simulink model "sm_wing_landing_gear"  (R2021b)
settings: Solver=ode45  StartTime=0  StopTime=10  RelTol=1e-4  AbsTol=1e-4  EnableMultiTasking=on
model workspace (MAT data in the model file):
  ddgrey = [0.15 0.15 0.15]
  dgrey = [0.3 0.3 0.3]
  grey = [0.5 0.5 0.5]
  lgrey = [0.7 0.7 0.7]
  rho_alum = 2700
undefined symbols (not defined in the file): sigbuilder_block, X, Y, Z
libraries: sm_lib x59, sm_wing_landing_gear_lib x45, nesl_utility x7, simulink x2
(part 3 of 3)

== system sm_wing_landing_gear/Wing Landing Gear/Main Column/Main Column/Art Links Bracket Housing ==
  Annular Cylinder : sm_wing_landing_gear_lib/Annular Cylinder  Ro=Ro  Ri=Ri  L=L  rho=rho  clr=clr  opc=1
      settings: SourceProductBaseCode=MS
  Left Side Transform : sm_lib/Frames and Transforms/Rigid Transform  TranslationMethod=Cylindrical  TranslationStandardOffset=0  TranslationLengthUnit=cm  TranslationStandardAxis=-Y  TranslationCartesianOffset=[0 0 0]  TranslationROffset=Ro  TranslationROffsetUnits=cm  TranslationZOffset=L/2  TranslationZOffsetUnits=cm  TranslationThetaOffset=-90  TranslationThetaOffsetUnits=deg  RotationMethod=AlignedAxes  RotationAngleUnits=deg  RotationStandardAxis=+Z  RotationAngle=0  RotationArbitraryAxis=[0 0 1]  FollAlignAxisA=+X  BaseAlignAxisA=-Y  FollAlignAxisB=+Y  BaseAlignAxisB=+X  RotationSequenceAxes=FollowerAxes  RotationSequence=XYX  RotationSequenceAngles=[0 0 0]  RotationSequenceAnglesUnits=deg  RotationMatrix=[1 0 0; 0 1 0; 0 0 1]
  Right Side Transform : sm_lib/Frames and Transforms/Rigid Transform  TranslationMethod=Cylindrical  TranslationStandardOffset=0  TranslationLengthUnit=cm  TranslationStandardAxis=-Y  TranslationCartesianOffset=[0 0 0]  TranslationROffset=Ro  TranslationROffsetUnits=cm  TranslationZOffset=L/2  TranslationZOffsetUnits=cm  TranslationThetaOffset=90  TranslationThetaOffsetUnits=deg  RotationMethod=AlignedAxes  RotationAngleUnits=deg  RotationStandardAxis=+Z  RotationAngle=0  RotationArbitraryAxis=[0 0 1]  FollAlignAxisA=+X  BaseAlignAxisA=+Y  FollAlignAxisB=+Y  BaseAlignAxisB=-X  RotationSequenceAxes=FollowerAxes  RotationSequence=XYX  RotationSequenceAngles=[0 0 0]  RotationSequenceAnglesUnits=deg  RotationMatrix=[1 0 0; 0 1 0; 0 0 1]
  T : PMIOPort  Side=Right
  L : PMIOPort  Port=2  Side=Left
  B : PMIOPort  Port=3  Side=Left
  R : PMIOPort  Port=4  Side=Left
  connections:
  Left Side Transform/RConn1 -- L/RConn1
  T/RConn1 -- Annular Cylinder/RConn1
  Right Side Transform/RConn1 -- R/RConn1
  Left Side Transform/LConn1 -- Right Side Transform/LConn1 -- Annular Cylinder/LConn1 -- B/RConn1

== system sm_wing_landing_gear/Wing Landing Gear/Main Column/Main Column/Main Actuator Bracket Housing ==
  Annular Cylinder : sm_wing_landing_gear_lib/Annular Cylinder  Ro=Ro  Ri=Ri  L=L  rho=rho  clr=clr  opc=1
      settings: SourceProductBaseCode=MS
  Left Side Transform : sm_lib/Frames and Transforms/Rigid Transform  TranslationMethod=Cylindrical  TranslationStandardOffset=0  TranslationLengthUnit=cm  TranslationStandardAxis=-Y  TranslationCartesianOffset=[0 0 0]  TranslationROffset=Ro  TranslationROffsetUnits=cm  TranslationZOffset=L/2  TranslationZOffsetUnits=cm  TranslationThetaOffset=180  TranslationThetaOffsetUnits=deg  RotationMethod=AlignedAxes  RotationAngleUnits=deg  RotationStandardAxis=+Z  RotationAngle=0  RotationArbitraryAxis=[0 0 1]  FollAlignAxisA=+X  BaseAlignAxisA=-X  FollAlignAxisB=+Y  BaseAlignAxisB=-Y  RotationSequenceAxes=FollowerAxes  RotationSequence=XYX  RotationSequenceAngles=[0 0 0]  RotationSequenceAnglesUnits=deg  RotationMatrix=[1 0 0; 0 1 0; 0 0 1]
  Right Side Transform : sm_lib/Frames and Transforms/Rigid Transform  TranslationMethod=Cylindrical  TranslationStandardOffset=0  TranslationLengthUnit=cm  TranslationStandardAxis=-Y  TranslationCartesianOffset=[0 0 0]  TranslationROffset=Ro  TranslationROffsetUnits=cm  TranslationZOffset=L/2  TranslationZOffsetUnits=cm  TranslationThetaOffset=0  TranslationThetaOffsetUnits=deg  RotationMethod=None  RotationAngleUnits=deg  RotationStandardAxis=+Z  RotationAngle=0  RotationArbitraryAxis=[0 0 1]  FollAlignAxisA=+X  BaseAlignAxisA=+Y  FollAlignAxisB=+Y  BaseAlignAxisB=-X  RotationSequenceAxes=FollowerAxes  RotationSequence=XYX  RotationSequenceAngles=[0 0 0]  RotationSequenceAnglesUnits=deg  RotationMatrix=[1 0 0; 0 1 0; 0 0 1]
  T : PMIOPort  Side=Right
  L : PMIOPort  Port=2  Side=Left
  B : PMIOPort  Port=3  Side=Left
  R : PMIOPort  Port=4  Side=Left
  connections:
  B/RConn1 -- Annular Cylinder/LConn1 -- Right Side Transform/LConn1 -- Left Side Transform/LConn1
  Right Side Transform/RConn1 -- R/RConn1
  T/RConn1 -- Annular Cylinder/RConn1
  Left Side Transform/RConn1 -- L/RConn1

== system sm_wing_landing_gear/Wing Landing Gear/Main Column/Main Column/Main Column Bottom Cylinder ==
  Annular Cylinder : sm_wing_landing_gear_lib/Annular Cylinder  Ro=Ro  Ri=Ri  L=L  rho=rho  clr=clr  opc=1
      settings: SourceProductBaseCode=MS
  Side Transform : sm_lib/Frames and Transforms/Rigid Transform  TranslationMethod=Cylindrical  TranslationStandardOffset=0  TranslationLengthUnit=cm  TranslationStandardAxis=+X  TranslationCartesianOffset=[ 0 0]  TranslationROffset=Ro  TranslationROffsetUnits=cm  TranslationZOffset=Oh  TranslationZOffsetUnits=cm  TranslationThetaOffset=Ah  TranslationThetaOffsetUnits=deg  RotationMethod=StandardAxis  RotationAngleUnits=deg  RotationStandardAxis=+Z  RotationAngle=Ah  RotationArbitraryAxis=[0 0 1]  FollAlignAxisA=+X  BaseAlignAxisA=+Y  FollAlignAxisB=+Y  BaseAlignAxisB=+Z  RotationSequenceAxes=FollowerAxes  RotationSequence=XYX  RotationSequenceAngles=[0 0 0]  RotationSequenceAnglesUnits=deg  RotationMatrix=[1 0 0; 0 1 0; 0 0 1]
  B : PMIOPort  Side=Left
  T : PMIOPort  Port=2  Side=Right
  D : PMIOPort  Port=3  Side=Left
  connections:
  Side Transform/LConn1 -- Annular Cylinder/LConn1 -- B/RConn1
  Annular Cylinder/RConn1 -- T/RConn1
  Side Transform/RConn1 -- D/RConn1

== system sm_wing_landing_gear/Wing Landing Gear/Main Column/Main Column/Main Column Top Cylinder ==
  Annular Cylinder : sm_wing_landing_gear_lib/Annular Cylinder  Ro=Ro  Ri=Ri  L=L  rho=rho  clr=clr  opc=1
      settings: SourceProductBaseCode=MS
  B : PMIOPort  Side=Left
  T : PMIOPort  Port=2  Side=Right
  connections:
  Annular Cylinder/RConn1 -- T/RConn1
  B/RConn1 -- Annular Cylinder/LConn1

== system sm_wing_landing_gear/Wing Landing Gear/Main Column/Main Column/Piston  ==
  Flange : sm_wing_landing_gear_lib/Annular Cylinder  Ro=Rf  Ri=Ri  L=Tf  rho=rho_alum  clr=clr  opc=1
      settings: SourceProductBaseCode=MS
  Piston : sm_wing_landing_gear_lib/Annular Cylinder  Ro=Ro  Ri=Ri  L=L  rho=rho_alum  clr=clr  opc=1
      settings: SourceProductBaseCode=MS
  B : PMIOPort  Side=Right
  T : PMIOPort  Port=2  Side=Left
  connections:
  B/RConn1 -- Flange/LConn1
  Piston/RConn1 -- T/RConn1
  Flange/RConn1 -- Piston/LConn1

== system sm_wing_landing_gear/Wing Landing Gear/Main Column/Main Column/Spherical Cup and Holder ==
  Cup : Subsystem  mask{Rb=Rci, Ro=Rco, T=2, A=210, Cc=cclr}
      mask prompts: Rb "Ball radius:"; Ro "Cup outer radius:"; T "Strip thickness:"; A "Cup angle:"; Cc "Color:"
      mask init:
      | theta = (linspace(-(A/2+90),(A/2-90),A+1)*pi/180)';
      | cup_profile = [Ro*cos(theta) Ro*sin(theta)];
      | theta = (linspace((A/2-90),-(A/2+90),A+1)*pi/180)';
      | cup_profile = vertcat(cup_profile,[Rb*cos(theta) Rb*sin(theta)]);
  Holder Half A : sm_lib/Body Elements/Extruded Solid  GraphicAmbientColor=[0.5 0.0 0.0 1.0]  BasedOnType=Density  CenterOfMass=[0 0 0]  CenterOfMassUnits=m  GraphicDiffuseColor=hclr  ExportConvexHullGeometry=off  ExtrusionCrossSection=hinge_sec_a  ExtrusionCrossSectionUnits=cm  Density=rho  DensityUnits=kg/(m^3)  DoExposeReferenceFrame=on  GraphicEmissiveColor=[0.0 0.0 0.0 1.0]  ExportEntireGeometry=off  ExtrusionLength=Hh  ExtrusionLengthUnits=cm  ExtrusionType=General  SerializedFrames=<Frames/>  MarkerShape=Sphere  MarkerSize=10  GraphicType=FromGeometry  InertiaType=CalculateFromGeometry  Mass=1  MassUnits=kg  MomentsOfInertia=[1 1 1]  MomentsOfInertiaUnits=kg*m^2  PolygonNumSides=3  GraphicOpacity=1.0  PolygonOuterRadius=1  PolygonOuterRadiusUnits=m  ProductsOfInertia=[0 0 0]  ProductsOfInertiaUnits=kg*m^2  GraphicShininess=75  GraphicSpecularColor=[0.5 0.5 0.5 1.0]  GraphicVisPropType=SimpleVisualProperties
  Holder Half B : sm_lib/Body Elements/Extruded Solid  GraphicAmbientColor=[0.5 0.0 0.0 1.0]  BasedOnType=Density  CenterOfMass=[0 0 0]  CenterOfMassUnits=m  GraphicDiffuseColor=hclr  ExportConvexHullGeometry=off  ExtrusionCrossSection=hinge_sec_b  ExtrusionCrossSectionUnits=cm  Density=rho  DensityUnits=kg/(m^3)  DoExposeReferenceFrame=on  GraphicEmissiveColor=[0.0 0.0 0.0 1.0]  ExportEntireGeometry=off  ExtrusionLength=Hh  ExtrusionLengthUnits=cm  ExtrusionType=General  SerializedFrames=<Frames/>  MarkerShape=Sphere  MarkerSize=10  GraphicType=FromGeometry  InertiaType=CalculateFromGeometry  Mass=1  MassUnits=kg  MomentsOfInertia=[1 1 1]  MomentsOfInertiaUnits=kg*m^2  PolygonNumSides=3  GraphicOpacity=1.0  PolygonOuterRadius=1  PolygonOuterRadiusUnits=m  ProductsOfInertia=[0 0 0]  ProductsOfInertiaUnits=kg*m^2  GraphicShininess=75  GraphicSpecularColor=[0.5 0.5 0.5 1.0]  GraphicVisPropType=SimpleVisualProperties
  Holder-Cup Transform : sm_lib/Frames and Transforms/Rigid Transform  TranslationMethod=Cartesian  TranslationStandardOffset=0  TranslationLengthUnit=cm  TranslationStandardAxis=+X  TranslationCartesianOffset=[Oh 0 Hh/2]  TranslationROffset=0  TranslationROffsetUnits=m  TranslationZOffset=0  TranslationZOffsetUnits=m  TranslationThetaOffset=0  TranslationThetaOffsetUnits=deg  RotationMethod=None  RotationAngleUnits=deg  RotationStandardAxis=+Z  RotationAngle=0  RotationArbitraryAxis=[0 0 1]  FollAlignAxisA=+X  BaseAlignAxisA=+Y  FollAlignAxisB=+Y  BaseAlignAxisB=+Z  RotationSequenceAxes=FollowerAxes  RotationSequence=XYX  RotationSequenceAngles=[0 0 0]  RotationSequenceAnglesUnits=deg  RotationMatrix=[1 0 0; 0 1 0; 0 0 1]
  S : PMIOPort  Side=Right
  B : PMIOPort  Port=2  Side=Left
  connections:
  B/RConn1 -- Holder Half A/RConn1 -- Holder-Cup Transform/LConn1 -- Holder Half B/RConn1
  Holder-Cup Transform/RConn1 -- Cup/LConn1
  Cup/RConn1 -- S/RConn1

== system sm_wing_landing_gear/Wing Landing Gear/Main Column Locking Mechanism/Side Stay Linkage/Peg and Ball ==
  Ball : sm_lib/Body Elements/Spherical Solid  GraphicAmbientColor=[0.5 0.0 0.0 1.0]  BasedOnType=Density  CenterOfMass=[0 0 0]  CenterOfMassUnits=m  GraphicDiffuseColor=clr  Density=rho  DensityUnits=kg/(m^3)  DoExposeReferenceFrame=on  GraphicEmissiveColor=[0.0 0.0 0.0 1.0]  ExportEntireGeometry=off  SerializedExposedGeometries=<ExposedGeometries/>  SerializedFrames=<Frames/>  MarkerShape=Sphere  MarkerSize=10  GraphicType=FromGeometry  InertiaType=CalculateFromGeometry  Mass=1  MassUnits=kg  MomentsOfInertia=[1 1 1]  MomentsOfInertiaUnits=kg*m^2  GraphicOpacity=1.0  ProductsOfInertia=[0 0 0]  ProductsOfInertiaUnits=kg*m^2  GraphicShininess=75  GraphicSpecularColor=[0.5 0.5 0.5 1.0]  SphereRadius=Rb  SphereRadiusUnits=cm  GraphicVisPropType=SimpleVisualProperties
  Base-Peg Transform : sm_lib/Frames and Transforms/Rigid Transform  TranslationMethod=StandardAxis  TranslationStandardOffset=Lp/2  TranslationLengthUnit=cm  TranslationStandardAxis=+Z  TranslationCartesianOffset=[0 0 0]  TranslationROffset=0  TranslationROffsetUnits=m  TranslationZOffset=0  TranslationZOffsetUnits=m  TranslationThetaOffset=0  TranslationThetaOffsetUnits=deg  RotationMethod=None  RotationAngleUnits=deg  RotationStandardAxis=+Z  RotationAngle=0  RotationArbitraryAxis=[0 0 1]  FollAlignAxisA=+Z  BaseAlignAxisA=+X  FollAlignAxisB=+X  BaseAlignAxisB=-Z  RotationSequenceAxes=FollowerAxes  RotationSequence=XYX  RotationSequenceAngles=[0 0 0]  RotationSequenceAnglesUnits=deg  RotationMatrix=[1 0 0; 0 1 0; 0 0 1]
  Peg : sm_lib/Body Elements/Cylindrical Solid  GraphicAmbientColor=[0.5 0.0 0.0 1.0]  BasedOnType=Density  CenterOfMass=[0 0 0]  CenterOfMassUnits=m  GraphicDiffuseColor=clr  CylinderLength=Lp  CylinderLengthUnits=cm  CylinderRadius=Rp  CylinderRadiusUnits=cm  Density=rho  DensityUnits=kg/(m^3)  DoExposeReferenceFrame=on  GraphicEmissiveColor=[0.0 0.0 0.0 1.0]  ExportEntireGeometry=off  SerializedFrames=<Frames/>  MarkerShape=Sphere  MarkerSize=10  GraphicType=FromGeometry  InertiaType=CalculateFromGeometry  Mass=1  MassUnits=kg  MomentsOfInertia=[1 1 1]  MomentsOfInertiaUnits=kg*m^2  GraphicOpacity=1.0  ProductsOfInertia=[0 0 0]  ProductsOfInertiaUnits=kg*m^2  GraphicShininess=75  GraphicSpecularColor=[0.5 0.5 0.5 1.0]  GraphicVisPropType=SimpleVisualProperties
  Peg-Ball Transform : sm_lib/Frames and Transforms/Rigid Transform  TranslationMethod=StandardAxis  TranslationStandardOffset=Lp/2  TranslationLengthUnit=cm  TranslationStandardAxis=+Z  TranslationCartesianOffset=[0 0 0]  TranslationROffset=0  TranslationROffsetUnits=m  TranslationZOffset=0  TranslationZOffsetUnits=m  TranslationThetaOffset=0  TranslationThetaOffsetUnits=deg  RotationMethod=None  RotationAngleUnits=deg  RotationStandardAxis=+Z  RotationAngle=0  RotationArbitraryAxis=[0 0 1]  FollAlignAxisA=+Z  BaseAlignAxisA=+X  FollAlignAxisB=+X  BaseAlignAxisB=-Z  RotationSequenceAxes=FollowerAxes  RotationSequence=XYX  RotationSequenceAngles=[0 0 0]  RotationSequenceAnglesUnits=deg  RotationMatrix=[1 0 0; 0 1 0; 0 0 1]
  F : PMIOPort  Side=Right
  B : PMIOPort  Port=2  Side=Left
  connections:
  Base-Peg Transform/LConn1 -- B/RConn1
  Ball/RConn1 -- F/RConn1 -- Peg-Ball Transform/RConn1
  Base-Peg Transform/RConn1 -- Peg-Ball Transform/LConn1 -- Peg/RConn1

== system sm_wing_landing_gear/Wing Landing Gear/Main Column/Main Column/Spherical Cup and Holder/Cup ==
  Base-Center Transform : sm_lib/Frames and Transforms/Rigid Transform  TranslationMethod=StandardAxis  TranslationStandardOffset=Ro  TranslationLengthUnit=cm  TranslationStandardAxis=+Z  TranslationCartesianOffset=[0 0 0]  TranslationROffset=[]  TranslationROffsetUnits=m  TranslationZOffset=[]  TranslationZOffsetUnits=m  TranslationThetaOffset=[]  TranslationThetaOffsetUnits=deg  RotationMethod=None  RotationAngleUnits=deg  RotationStandardAxis=+X  RotationAngle=[]  RotationArbitraryAxis=[]  FollAlignAxisA=+X  BaseAlignAxisA=+Y  FollAlignAxisB=+Y  BaseAlignAxisB=+Z  RotationSequenceAxes=FollowerAxes  RotationSequence=XYX  RotationSequenceAngles=[0 0 0]  RotationSequenceAnglesUnits=deg  RotationMatrix=[1 0 0; 0 1 0; 0 0 1]
  Center-Strip A Transform : sm_lib/Frames and Transforms/Rigid Transform  TranslationMethod=None  TranslationStandardOffset=0  TranslationLengthUnit=m  TranslationStandardAxis=+X  TranslationCartesianOffset=[0 0 0]  TranslationROffset=[]  TranslationROffsetUnits=m  TranslationZOffset=[]  TranslationZOffsetUnits=m  TranslationThetaOffset=[]  TranslationThetaOffsetUnits=deg  RotationMethod=AlignedAxes  RotationAngleUnits=deg  RotationStandardAxis=+X  RotationAngle=[]  RotationArbitraryAxis=[]  FollAlignAxisA=+Y  BaseAlignAxisA=+Z  FollAlignAxisB=+Z  BaseAlignAxisB=-Y  RotationSequenceAxes=FollowerAxes  RotationSequence=XYX  RotationSequenceAngles=[0 0 0]  RotationSequenceAnglesUnits=deg  RotationMatrix=[1 0 0; 0 1 0; 0 0 1]
  Center-Strip B Transform : sm_lib/Frames and Transforms/Rigid Transform  TranslationMethod=None  TranslationStandardOffset=0  TranslationLengthUnit=m  TranslationStandardAxis=+X  TranslationCartesianOffset=[0 0 0]  TranslationROffset=[]  TranslationROffsetUnits=m  TranslationZOffset=[]  TranslationZOffsetUnits=m  TranslationThetaOffset=[]  TranslationThetaOffsetUnits=deg  RotationMethod=AlignedAxes  RotationAngleUnits=deg  RotationStandardAxis=+X  RotationAngle=[]  RotationArbitraryAxis=[]  FollAlignAxisA=+Z  BaseAlignAxisA=+X  FollAlignAxisB=+Y  BaseAlignAxisB=+Z  RotationSequenceAxes=FollowerAxes  RotationSequence=XYX  RotationSequenceAngles=[0 0 0]  RotationSequenceAnglesUnits=deg  RotationMatrix=[1 0 0; 0 1 0; 0 0 1]
  Cup Strip A : sm_lib/Body Elements/Extruded Solid  GraphicAmbientColor=[0.5 0.0 0.0 1.0]  BasedOnType=Density  CenterOfMass=[]  CenterOfMassUnits=m  GraphicDiffuseColor=Cc  ExportConvexHullGeometry=off  ExtrusionCrossSection=cup_profile  ExtrusionCrossSectionUnits=cm  Density=rho  DensityUnits=kg/(m^3)  DoExposeReferenceFrame=on  GraphicEmissiveColor=[0.0 0.0 0.0 1.0]  ExportEntireGeometry=off  ExtrusionLength=T  ExtrusionLengthUnits=cm  ExtrusionType=General  SerializedFrames=<Frames/>  MarkerShape=Sphere  MarkerSize=10  GraphicType=FromGeometry  InertiaType=CalculateFromGeometry  Mass=[]  MassUnits=kg  MomentsOfInertia=[]  MomentsOfInertiaUnits=kg*m^2  PolygonNumSides=[]  GraphicOpacity=1  PolygonOuterRadius=[]  PolygonOuterRadiusUnits=m  ProductsOfInertia=[]  ProductsOfInertiaUnits=kg*m^2  GraphicShininess=64.0  GraphicSpecularColor=[0.8 0.8 0.8 1.0]  GraphicVisPropType=SimpleVisualProperties
  Cup Strip B : sm_lib/Body Elements/Extruded Solid  GraphicAmbientColor=[0.5 0.0 0.0 1.0]  BasedOnType=Density  CenterOfMass=[]  CenterOfMassUnits=m  GraphicDiffuseColor=Cc  ExportConvexHullGeometry=off  ExtrusionCrossSection=cup_profile  ExtrusionCrossSectionUnits=cm  Density=rho  DensityUnits=kg/(m^3)  DoExposeReferenceFrame=on  GraphicEmissiveColor=[0.0 0.0 0.0 1.0]  ExportEntireGeometry=off  ExtrusionLength=T  ExtrusionLengthUnits=cm  ExtrusionType=General  SerializedFrames=<Frames/>  MarkerShape=Sphere  MarkerSize=10  GraphicType=FromGeometry  InertiaType=CalculateFromGeometry  Mass=[]  MassUnits=kg  MomentsOfInertia=[]  MomentsOfInertiaUnits=kg*m^2  PolygonNumSides=[]  GraphicOpacity=1  PolygonOuterRadius=[]  PolygonOuterRadiusUnits=m  ProductsOfInertia=[]  ProductsOfInertiaUnits=kg*m^2  GraphicShininess=64.0  GraphicSpecularColor=[0.8 0.8 0.8 1.0]  GraphicVisPropType=SimpleVisualProperties
  B : PMIOPort  Tag=PMCPort  Side=Left
  C : PMIOPort  Tag=PMCPort  Port=2  Side=Right
  connections:
  B/RConn1 -- Base-Center Transform/LConn1
  Base-Center Transform/RConn1 -- Center-Strip A Transform/LConn1 -- Center-Strip B Transform/LConn1 -- C/RConn1
  Cup Strip A/RConn1 -- Center-Strip A Transform/RConn1
  Cup Strip B/RConn1 -- Center-Strip B Transform/RConn1
